simulink model "kin_lin_dyn_FSMRAC_lin2"  (R2017b)
settings: Solver=ode45  StartTime=0.0  StopTime=25  RelTol=1e-3
values from neighbouring files (symbols this model uses):
  act_theta1 = 0.021281    [FSMRAC_lin2.m]
  act_theta2 = 0.02017    [FSMRAC_lin2.m]
  act_theta3 = 1.2e-4    (= 0.00012)    [FSMRAC_lin2.m]
  act_theta4 = 1.0236    [FSMRAC_lin2.m]
  act_theta5 = 1.0438e-4    (= 0.00010438)    [FSMRAC_lin2.m]
  act_theta6 = 1.00271    [FSMRAC_lin2.m]
  alpha = 1    [FSMRAC_lin2.m]
  am = 5    [FSMRAC_lin2.m]
  Am = -am*eye(2)    [FSMRAC_lin2.m]
  Bm = eye(2)    [FSMRAC_lin2.m]
  Cm = eye(2)    [FSMRAC_lin2.m]
  disturbance = 1    [FSMRAC_lin2.m]
  Dm = zeros(2,2)    [FSMRAC_lin2.m]
  Gamma = eye(8)    [FSMRAC_lin2.m]
  P0 = eye(6)    [FSMRAC_lin2.m]
  P_lyap = lyap(Am,Q)    [FSMRAC_lin2.m]
  phi_init = pi/2    (= 1.57079632679)    [FSMRAC_lin2.m]
  R = 2    [FSMRAC_lin2.m]    (also in kinsim.m)
  theta0_c = ones(1,8)    [FSMRAC_lin2.m]
  theta0_m = ones(1,6)    [FSMRAC_lin2.m]
  x_init = 2    [FSMRAC_lin2.m]
  y_init = 0    [FSMRAC_lin2.m]
undefined symbols (not defined in the file or in its folder): magnitude
libraries: simulink_extras x8
settings Model: Creator=nadimkhairallah  LastModifiedBy=nadimkhairallah

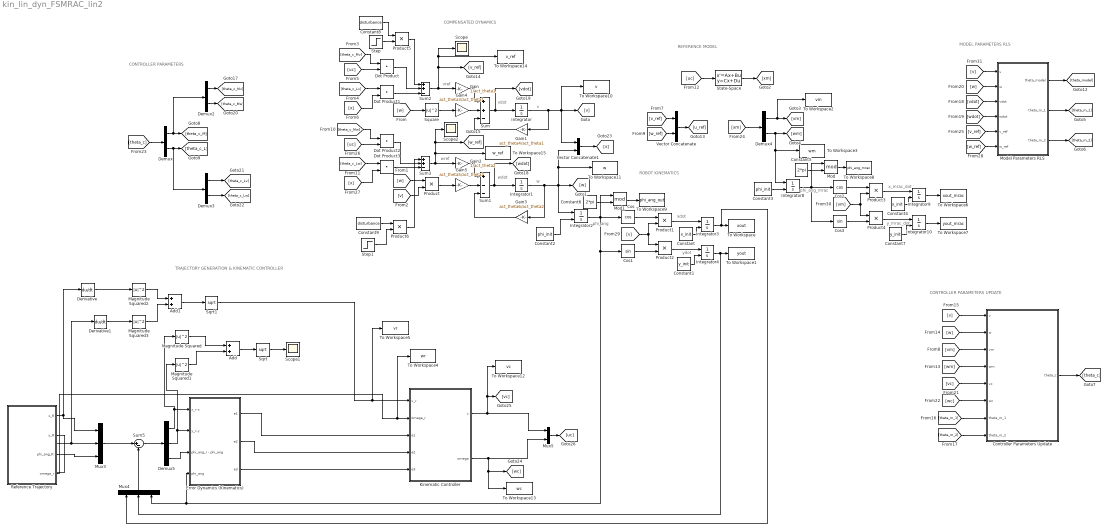
== system kin_lin_dyn_FSMRAC_lin2 ==
  note: ROBOT KINEMATICS
  note: xdot
  note: phi_ang
  note: REFERENCE MODEL
  note: COMPENSATED DYNAMICS
  note: TRAJECTORY GENERATION & KINEMATIC CONTROLLER
  note: CONTROLLER PARAMETERS
  note: w
  note: v
  note: vdot
  note: vref
  note: wdot
  note: wref
  note: CONTROLLER PARAMETERS UPDATE
  note: MODEL PARAMETERS RLS
  note: ydot
  note: y_mrac_dot
  note: x_mrac_dot
  note: phi_ang_mrac
  Add : Sum
  Add1 : Sum
  Constant : Constant  Value=x_init
  Constant1 : Constant  Value=y_init
  Constant2 : Constant  Value=phi_init
  Constant3 : Constant  Value=phi_init
  Constant4 : Constant  Value=x_init
  Constant5 : Constant  Value=2*pi
  Constant6 : Constant  Value=2*pi
  Constant7 : Constant  Value=y_init
  Constant8 : Constant  Value=disturbance
  Constant9 : Constant  Value=disturbance
  Controller Parameters Update : Subsystem
  Cos : Trigonometry  Operator=cos
  Cos1 : Trigonometry
  Cos2 : Trigonometry  Operator=cos
  Cos3 : Trigonometry
  Demux{,2..4} (4 alike) : Demux  Outputs=2
  Demux5 : Demux  Outputs=3
  Derivative : Derivative
  Derivative1 : Derivative
  Dot Product{,1..3} (4 alike) : DotProduct  InputSameDT=on  OutDataTypeStr=Inherit: Inherit via internal rule
  Error Dynamics (Kinematics) : Subsystem
  Gain : Gain  Gain=1/act_theta1
  Gain1 : Gain  Gain=act_theta4/act_theta1
  Gain2 : Gain  Gain=1/act_theta2
  Gain3 : Gain  Gain=act_theta6/act_theta2
  Gain4 : Gain  Gain=act_theta3/act_theta1
  Gain5 : Gain  Gain=act_theta5/act_theta2
  Integrator : Integrator
  Integrator1 : Integrator
  Integrator{2..4,8..10} (6 alike) : Integrator  InitialConditionSource=external
  Kinematic Controller : Subsystem
  Magnitude Squared{,1..3} (4 alike) : Math  Operator=magnitude^2  SaturateOnIntegerOverflow=on
  Mod : Math  Operator=mod  SaturateOnIntegerOverflow=on
  Mod1 : Math  Operator=mod  SaturateOnIntegerOverflow=on
  Model Parameters RLS : Subsystem
  Mux3 : Mux  Inputs=3
  Mux4 : Mux  Inputs=3
  Mux5 : Mux  Inputs=2
  Product{,1..6} (7 alike) : Product
  Reference Trajectory : Subsystem
  Scope : Scope
  Scope1 : Scope
  Scope2 : Scope
  Sqrt : Sqrt  SaturateOnIntegerOverflow=on
  Sqrt1 : Sqrt  SaturateOnIntegerOverflow=on
  Square : Math  Operator=magnitude^2  RndMeth=Zero  SaturateOnIntegerOverflow=on
  State-Space : StateSpace  A=Am  B=Bm  C=Cm  D=Dm  InitialCondition=0
  Step : Step  Time=15  After=0.5  SampleTime=0
  Step1 : Step  Time=10  After=0.5  SampleTime=0
  Sum : Sum  Inputs=++-
  Sum1 : Sum  Inputs=+--
  Sum2 : Sum  Inputs=++-
  Sum3 : Sum  Inputs=++-
  Sum5 : Sum  Inputs=|+-
  To Workspace : ToWorkspace  VariableName=xout  SampleTime=-1
      settings: Save2DSignal=2-D array (concatenate along first dimension)
  To Workspace1 : ToWorkspace  VariableName=yout  SampleTime=-1
      settings: Save2DSignal=2-D array (concatenate along first dimension)
  To Workspace10 : ToWorkspace  VariableName=v  SampleTime=-1
  To Workspace11 : ToWorkspace  VariableName=w  SampleTime=-1
  To Workspace12 : ToWorkspace  VariableName=vc  SampleTime=-1
      settings: Save2DSignal=2-D array (concatenate along first dimension)
  To Workspace13 : ToWorkspace  VariableName=wc  SampleTime=-1
      settings: Save2DSignal=2-D array (concatenate along first dimension)
  To Workspace14 : ToWorkspace  VariableName=v_ref  SampleTime=-1
  To Workspace15 : ToWorkspace  VariableName=w_ref  SampleTime=-1
  To Workspace2 : ToWorkspace  VariableName=vm  SampleTime=-1
  To Workspace3 : ToWorkspace  VariableName=wm  SampleTime=-1
  To Workspace4 : ToWorkspace  VariableName=wr  SampleTime=-1
  To Workspace5 : ToWorkspace  VariableName=vr  SampleTime=-1
  To Workspace6 : ToWorkspace  VariableName=xout_mrac  SampleTime=-1
  To Workspace7 : ToWorkspace  VariableName=yout_mrac  SampleTime=-1
  To Workspace8 : ToWorkspace  VariableName=phi_ang_mrac  SampleTime=-1
  To Workspace9 : ToWorkspace  VariableName=phi_ang_out  SampleTime=-1
      settings: Save2DSignal=2-D array (concatenate along first dimension)
  Vector Concatenate : Concatenate
  Vector Concatenate1 : Concatenate
  wires:
  Gain/1 -> Sum/1
  Gain1/1 -> Sum/3
  Gain3/1 -> Sum1/3
  Gain2/1 -> Sum1/1
  [w] -> Square/1
  Gain4/1 -> Sum/2
  Square/1 -> Gain4/1
  Gain5/1 -> Sum1/2
  Product/1 -> Gain5/1
  [w] -> Product/1
  [v] -> Product/2
  [v] -> Controller Parameters Update/1(v)
  [w] -> Controller Parameters Update/2(w)
  [vm] -> Controller Parameters Update/3(vm)
  [wm] -> Controller Parameters Update/4(wm)
  [theta_m_1] -> Controller Parameters Update/7(theta_m_1)
  [theta_m_2] -> Controller Parameters Update/8(theta_m_2)
  [vc] -> Controller Parameters Update/5(vc)
  [wc] -> Controller Parameters Update/6(wc)
  Controller Parameters Update/1(theta_c) -> [theta_c]
  [theta_c] -> Demux/1
  Demux/1 -> [theta_c_M], Demux2/1
  Demux/2 -> Demux3/1, [theta_c_L]
  Demux2/1 -> [theta_c_Mv]
  Demux2/2 -> [theta_c_Mw]
  Demux3/1 -> [theta_c_Lv]
  Demux3/2 -> [theta_c_Lw]
  [theta_c_Mv] -> Dot Product/1
  [uc] -> Dot Product/2
  [theta_c_Lv] -> Dot Product1/1
  [x] -> Dot Product1/2
  [v_ref] -> Vector Concatenate/1
  Vector Concatenate/1 -> [u_ref]
  [x] -> Dot Product3/2
  [theta_c_Lw] -> Dot Product3/1
  [uc] -> Dot Product2/2
  [theta_c_Mw] -> Dot Product2/1
  [uc] -> State-Space/1
  State-Space/1 -> [xm]
  [xm] -> Demux4/1
  Demux4/1 -> To Workspace2/1, [vm]
  Demux4/2 -> Integrator8/1, To Workspace3/1, [wm]
  [w_ref] -> Vector Concatenate/2
  Vector Concatenate1/1 -> [x]
  [vdot] -> Model Parameters RLS/3("vdot ")
  Model Parameters RLS/1(theta_model) -> [theta_model]
  [w] -> Model Parameters RLS/2(w)
  [v] -> Model Parameters RLS/1(v)
  [wdot] -> Model Parameters RLS/4("wdot ")
  [v_ref] -> Model Parameters RLS/5(v_ref)
  Model Parameters RLS/2(theta_m_1) -> [theta_m_1]
  Model Parameters RLS/3(theta_m_2) -> [theta_m_2]
  [w_ref] -> Model Parameters RLS/6(w_ref)
  Integrator1/1 -> [w], Integrator2/1, To Workspace11/1, Vector Concatenate1/2, Gain3/1
  Sum/1 -> [vdot], Integrator/1
  Sum1/1 -> [wdot], Integrator1/1
  Sum2/1 -> Scope/1, To Workspace14/1, [v_ref], Gain/1
  Sum3/1 -> To Workspace15/1, [w_ref], Scope2/1, Gain2/1
  Cos/1 -> Product1/1
  [v] -> Product2/1, Product1/2
  Cos1/1 -> Product2/2
  Product1/1 -> Integrator3/1
  Product2/1 -> Integrator4/1
  Constant/1 -> Integrator3/2
  Constant1/1 -> Integrator4/2
  Constant2/1 -> Integrator2/2
  Magnitude Squared2/1 -> Add1/1
  Magnitude Squared3/1 -> Add1/2
  Reference Trajectory/3("phi_ang_R ") -> Mux3/3
  Derivative1/1 -> Magnitude Squared3/1
  Reference Trajectory/1("x_R ") -> Mux3/1, Derivative/1
  Integrator3/1 -> Mux4/1, To Workspace/1
  Mux3/1 -> Sum5/1
  Add/1 -> Sqrt/1
  Magnitude Squared1/1 -> Add/2
  Error Dynamics (Kinematics)/2(e2) -> Kinematic Controller/4(e2)
  Error Dynamics (Kinematics)/3(e3) -> Kinematic Controller/5(e3)
  Integrator4/1 -> Mux4/2, To Workspace1/1
  Sum5/1 -> Demux5/1
  Sqrt/1 -> Scope1/1
  Mux4/1 -> Sum5/2
  Magnitude Squared/1 -> Add/1
  Demux5/3 -> Error Dynamics (Kinematics)/3("phi_ang_r - phi_ang ")
  Reference Trajectory/4("omega_r ") -> To Workspace4/1, Kinematic Controller/2(omega_r)
  Integrator2/1 -> Mod1/1, Mux4/3, Error Dynamics (Kinematics)/4(phi_ang), Cos1/1, Cos/1
  Error Dynamics (Kinematics)/1(e1) -> Kinematic Controller/3(e1)
  Demux5/2 -> Magnitude Squared1/1, Error Dynamics (Kinematics)/2(y_r-y)
  Add1/1 -> Sqrt1/1
  Demux5/1 -> Magnitude Squared/1, Error Dynamics (Kinematics)/1("x_r-x ")
  Derivative/1 -> Magnitude Squared2/1
  Reference Trajectory/2("y_R ") -> Derivative1/1, Mux3/2
  Sqrt1/1 -> Kinematic Controller/1(v_r), To Workspace5/1
  Mux5/1 -> [uc]
  Kinematic Controller/2(omega) -> To Workspace13/1, [wc], Mux5/2
  Kinematic Controller/1(v) -> Mux5/1, To Workspace12/1, [vc]
  Cos3/1 -> Product4/2
  Cos2/1 -> Product3/1
  Constant3/1 -> Integrator8/2
  Constant7/1 -> Integrator10/2
  Integrator10/1 -> To Workspace7/1
  Product4/1 -> Integrator10/1
  [vm] -> Product3/2, Product4/1
  Constant4/1 -> Integrator9/2
  Product3/1 -> Integrator9/1
  Integrator9/1 -> To Workspace6/1
  Mod/1 -> To Workspace8/1
  Integrator8/1 -> Mod/1, Cos2/1, Cos3/1
  Constant5/1 -> Mod/2
  Constant6/1 -> Mod1/2
  Mod1/1 -> To Workspace9/1
  Integrator/1 -> [v], Vector Concatenate1/1, To Workspace10/1, Gain1/1
  Dot Product1/1 -> Sum2/3
  Dot Product/1 -> Sum2/2
  Dot Product3/1 -> Sum3/3
  Dot Product2/1 -> Sum3/2
  Step/1 -> Product5/2
  Constant8/1 -> Product5/1
  Product5/1 -> Sum2/1
  Constant9/1 -> Product6/1
  Step1/1 -> Product6/2
  Product6/1 -> Sum3/1

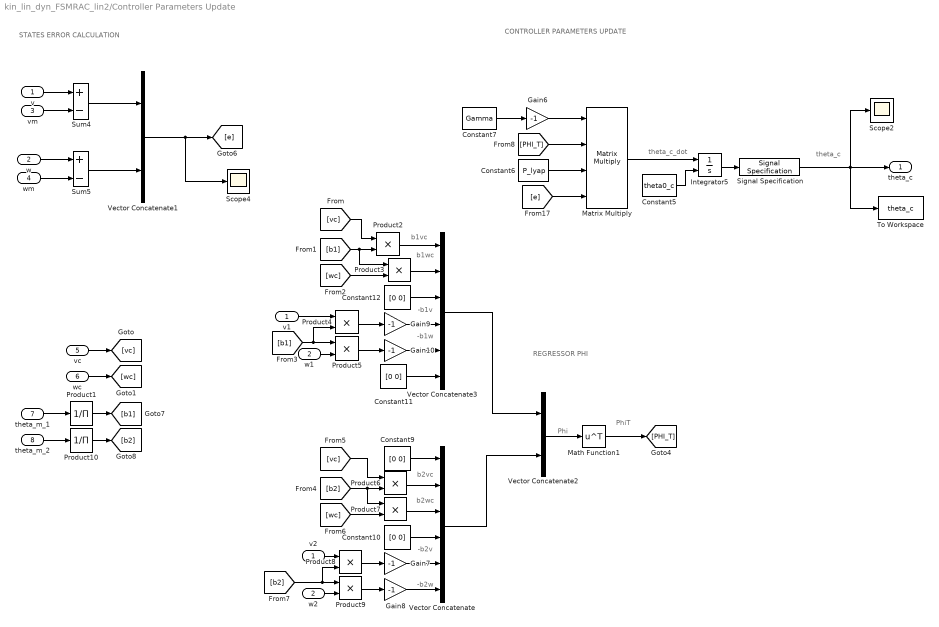
== system kin_lin_dyn_FSMRAC_lin2/Controller Parameters Update ==
  note: -b2v
  note: b2vc
  note: theta_c
  note: theta_c_dot
  note: STATES ERROR CALCULATION
  note: CONTROLLER PARAMETERS UPDATE
  note: PhiT
  note: REGRESSOR PHI
  note: Phi
  note: b2wc
  note: -b2w
  note: b1vc
  note: b1wc
  note: -b1v
  note: -b1w
  v : Inport
  w : Inport  Port=2
  vm : Inport  Port=3
  wm : Inport  Port=4
  vc : Inport  Port=5
  wc : Inport  Port=6
  theta_m_1 : Inport  Port=7
  theta_m_2 : Inport  Port=8
  Constant{9..12} (4 alike) : Constant  Value=[0 0]  VectorParams1D=off
  Constant5 : Constant  Value=theta0_c
  Constant6 : Constant  Value=P_lyap  VectorParams1D=off
  Constant7 : Constant  Value=Gamma  VectorParams1D=off
  Gain{6..10} (5 alike) : Gain  Gain=-1
  Integrator5 : Integrator  InitialConditionSource=external
  Math Function1 : Math  Operator=transpose  SaturateOnIntegerOverflow=on
  Matrix Multiply : Product  Inputs=4  Multiplication=Matrix(*)
  Product1 : Product  Inputs=/
  Product10 : Product  Inputs=/
  Product{2..9} (8 alike) : Product
  Scope2 : Scope
  Scope4 : Scope
  Signal Specification : SignalSpecification  Dimensions=8*1
  Sum4 : Sum  Inputs=+-
  Sum5 : Sum  Inputs=+-
  To Workspace : ToWorkspace  VariableName=theta_c  SampleTime=-1
      settings: Save2DSignal=2-D array (concatenate along first dimension)
  Vector Concatenate : Concatenate  NumInputs=6
  Vector Concatenate1 : Concatenate  Mode=Multidimensional array
  Vector Concatenate2 : Concatenate  Mode=Multidimensional array
  Vector Concatenate3 : Concatenate  NumInputs=6
  v1 : InportShadow
  v2 : InportShadow
  w1 : InportShadow  Port=2
  w2 : InportShadow  Port=2
  theta_c : Outport
  wires:
  Constant10/1 -> Vector Concatenate/4
  Gain8/1 -> Vector Concatenate/6
  Vector Concatenate2/1 -> Math Function1/1
  Gain6/1 -> Matrix Multiply/1
  Constant12/1 -> Vector Concatenate3/3
  Sum4/1 -> Vector Concatenate1/1
  [e] -> Matrix Multiply/4
  Constant11/1 -> Vector Concatenate3/6
  Constant6/1 -> Matrix Multiply/3
  Vector Concatenate3/1 -> Vector Concatenate2/1
  Math Function1/1 -> [PHI_T]
  Constant7/1 -> Gain6/1
  Sum5/1 -> Vector Concatenate1/2
  Gain10/1 -> Vector Concatenate3/5
  Gain9/1 -> Vector Concatenate3/4
  Matrix Multiply/1 -> Integrator5/1
  Constant5/1 -> Integrator5/2
  Vector Concatenate/1 -> Vector Concatenate2/2
  [PHI_T] -> Matrix Multiply/2
  Constant9/1 -> Vector Concatenate/1
  Vector Concatenate1/1 -> [e], Scope4/1
  Gain7/1 -> Vector Concatenate/5
  v/1 -> Sum4/1
  w/1 -> Sum5/1
  wm/1 -> Sum5/2
  vm/1 -> Sum4/2
  vc/1 -> [vc]
  wc/1 -> [wc]
  Product2/1 -> Vector Concatenate3/1
  [vc] -> Product2/1
  [b1] -> Product3/1, Product2/2
  Product3/1 -> Vector Concatenate3/2
  [wc] -> Product3/2
  Product4/1 -> Gain9/1
  Product5/1 -> Gain10/1
  v1/1 -> Product4/1
  [b1] -> Product4/2, Product5/1
  w1/1 -> Product5/2
  Product6/1 -> Vector Concatenate/2
  Product7/1 -> Vector Concatenate/3
  [b2] -> Product7/1, Product6/2
  [vc] -> Product6/1
  [wc] -> Product7/2
  Product8/1 -> Gain7/1
  Product9/1 -> Gain8/1
  v2/1 -> Product8/1
  [b2] -> Product8/2, Product9/1
  w2/1 -> Product9/2
  theta_m_2/1 -> Product10/1
  theta_m_1/1 -> Product1/1
  Product1/1 -> [b1]
  Product10/1 -> [b2]
  Integrator5/1 -> Signal Specification/1
  Signal Specification/1 -> To Workspace/1, Scope2/1, theta_c/1

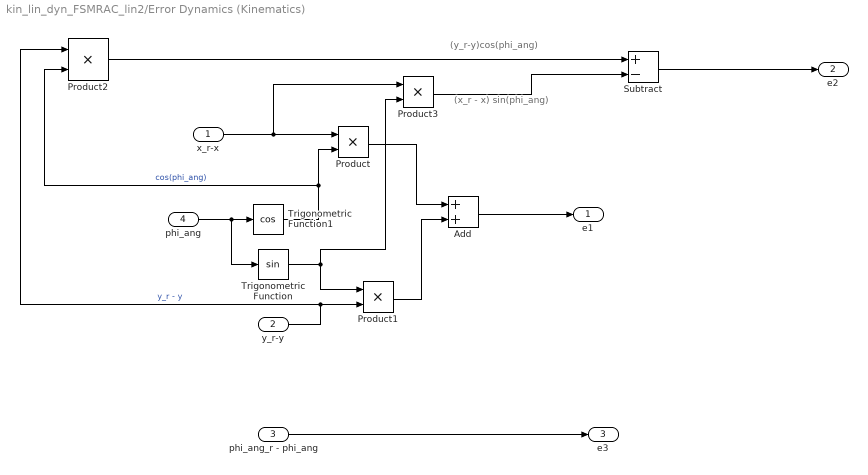
== system kin_lin_dyn_FSMRAC_lin2/Error Dynamics (Kinematics) ==
  note: (x_r - x) sin(phi_ang)
  note: (y_r-y)cos(phi_ang)
  "x_r-x " : Inport
  y_r-y : Inport  Port=2
  "phi_ang_r - phi_ang " : Inport  Port=3
  phi_ang : Inport  Port=4
  Add : Sum
  Product{,1..3} (4 alike) : Product
  Subtract : Sum  Inputs=+-
  Trigonometric Function : Trigonometry
  Trigonometric Function1 : Trigonometry  Operator=cos
  e1 : Outport  VectorParamsAs1DForOutWhenUnconnected=on
  e2 : Outport  Port=2  VectorParamsAs1DForOutWhenUnconnected=on
  e3 : Outport  Port=3  VectorParamsAs1DForOutWhenUnconnected=on
  wires:
  "x_r-x "/1 -> Product3/1, Product/1
  phi_ang/1 -> Trigonometric Function/1, Trigonometric Function1/1
  Trigonometric Function1/1 -> Product2/2, Product/2  "cos(phi_ang)"
  Trigonometric Function/1 -> Product3/2, Product1/1
  y_r-y/1 -> Product2/1, Product1/2  "y_r - y"
  "phi_ang_r - phi_ang "/1 -> e3/1
  Product1/1 -> Add/2
  Product/1 -> Add/1
  Add/1 -> e1/1
  Product2/1 -> Subtract/1
  Product3/1 -> Subtract/2
  Subtract/1 -> e2/1

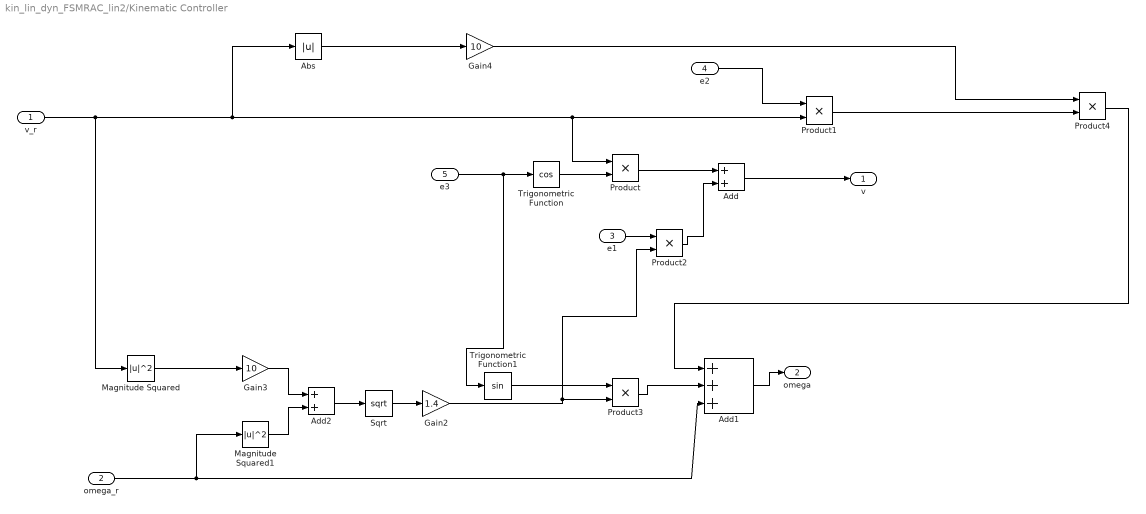
== system kin_lin_dyn_FSMRAC_lin2/Kinematic Controller ==
  v_r : Inport
  omega_r : Inport  Port=2
  e1 : Inport  Port=3
  e2 : Inport  Port=4
  e3 : Inport  Port=5
  Abs : Abs
  Add : Sum
  Add1 : Sum  Inputs=+++
  Add2 : Sum
  Gain2 : Gain  Gain=1.4
  Gain3 : Gain  Gain=10
  Gain4 : Gain  Gain=10
  Magnitude Squared : Math  Operator=magnitude^2  SaturateOnIntegerOverflow=on
  Magnitude Squared1 : Math  Operator=magnitude^2  SaturateOnIntegerOverflow=on
  Product{,1..4} (5 alike) : Product
  Sqrt : Sqrt  SaturateOnIntegerOverflow=on
  Trigonometric Function : Trigonometry  Operator=cos
  Trigonometric Function1 : Trigonometry
  v : Outport  VectorParamsAs1DForOutWhenUnconnected=on
  omega : Outport  Port=2  VectorParamsAs1DForOutWhenUnconnected=on
  wires:
  Trigonometric Function/1 -> Product/2
  v_r/1 -> Abs/1, Product/1, Product1/2, Magnitude Squared/1
  Product/1 -> Add/1
  e1/1 -> Product2/1
  Product2/1 -> Add/2
  Add/1 -> v/1
  Add1/1 -> omega/1
  Trigonometric Function1/1 -> Product3/1
  e3/1 -> Trigonometric Function1/1, Trigonometric Function/1
  omega_r/1 -> Add1/3, Magnitude Squared1/1
  Product3/1 -> Add1/2
  Product4/1 -> Add1/1
  e2/1 -> Product1/1
  Product1/1 -> Product4/2
  Magnitude Squared1/1 -> Add2/2
  Magnitude Squared/1 -> Gain3/1
  Gain3/1 -> Add2/1
  Add2/1 -> Sqrt/1
  Sqrt/1 -> Gain2/1
  Gain2/1 -> Product2/2, Product3/2
  Abs/1 -> Gain4/1
  Gain4/1 -> Product4/1

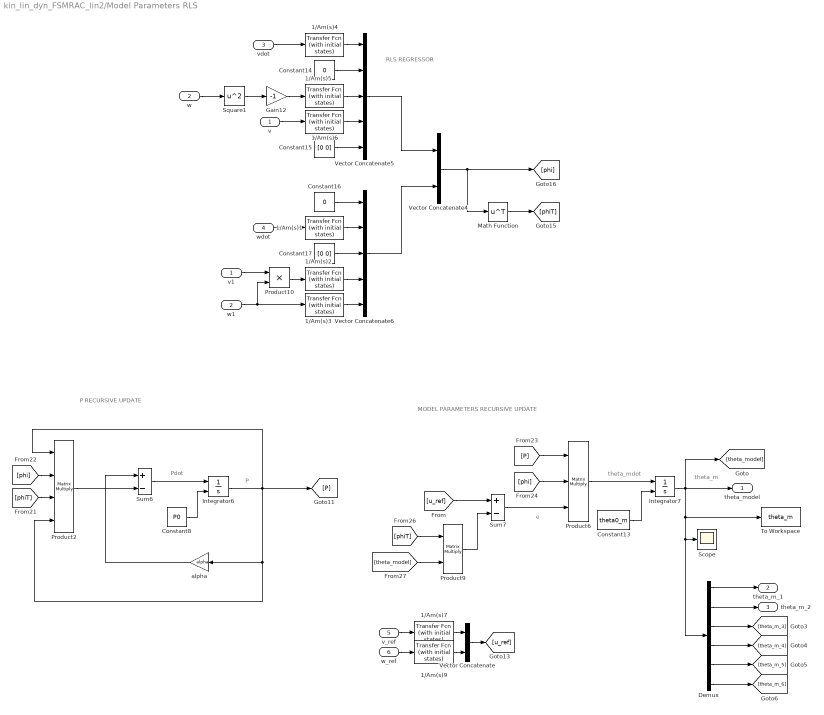
== system kin_lin_dyn_FSMRAC_lin2/Model Parameters RLS ==
  note: e
  note: theta_m
  note: theta_mdot
  note: P
  note: Pdot
  note: MODEL PARAMETERS RECURSIVE UPDATE
  note: P RECURSIVE UPDATE
  note: RLS REGRESSOR
  v : Inport  PortDimensions=1
  w : Inport  Port=2  PortDimensions=1
  "vdot " : Inport  Port=3  PortDimensions=1
  "wdot " : Inport  Port=4  PortDimensions=1
  v_ref : Inport  Port=5  PortDimensions=1
  w_ref : Inport  Port=6  PortDimensions=1
  1/Am(s){1..7,9} (8 alike) : simulink_extras/Additional Linear/Transfer Fcn (with initial states)  N=[1]  D=[1 2*am am^2]  X0=.5
  Constant13 : Constant  Value=theta0_m
  Constant14 : Constant  Value=0
  Constant15 : Constant  Value=[0 0]
  Constant16 : Constant  Value=0
  Constant17 : Constant  Value=[0 0]
  Constant8 : Constant  Value=P0
  Demux : Demux  Outputs=6
  Gain12 : Gain  Gain=-1
  Integrator6 : Integrator  InitialConditionSource=external  InitialCondition=P0
  Integrator7 : Integrator  InitialConditionSource=external  InitialCondition=P0
  Math Function : Math  Operator=transpose  SaturateOnIntegerOverflow=on
  Product10 : Product
  Product2 : Product  Inputs=4  Multiplication=Matrix(*)
  Product6 : Product  Inputs=3  Multiplication=Matrix(*)
  Product9 : Product  Multiplication=Matrix(*)
  Scope : Scope
  Square1 : Math  Operator=square  RndMeth=Zero  SaturateOnIntegerOverflow=on
  Sum6 : Sum  Inputs=+-
  Sum7 : Sum  Inputs=+-
  To Workspace : ToWorkspace  VariableName=theta_m  SampleTime=-1
  Vector Concatenate : Concatenate
  Vector Concatenate4 : Concatenate  Mode=Multidimensional array  ConcatenateDimension=2
  Vector Concatenate5 : Concatenate  NumInputs=5  ConcatenateDimension=2
  Vector Concatenate6 : Concatenate  NumInputs=5  ConcatenateDimension=2
  "alpha " : Gain  Gain=alpha
  v1 : InportShadow  PortDimensions=1
  w1 : InportShadow  Port=2  PortDimensions=1
  theta_model : Outport
  theta_m_1 : Outport  Port=2
  theta_m_2 : Outport  Port=3
  wires:
  Constant15/1 -> Vector Concatenate5/5
  Constant17/1 -> Vector Concatenate6/3
  1/Am(s)5/1 -> Vector Concatenate5/3
  1/Am(s)2/1 -> Vector Concatenate6/4
  Gain12/1 -> 1/Am(s)5/1
  Product10/1 -> 1/Am(s)2/1
  1/Am(s)3/1 -> Vector Concatenate6/5
  Vector Concatenate5/1 -> Vector Concatenate4/1
  1/Am(s)4/1 -> Vector Concatenate5/1
  [phiT] -> Product9/1
  [theta_model] -> Product9/2
  Constant13/1 -> Integrator7/2
  Integrator6/1 -> Product2/4, "alpha "/1, [P], Product2/1
  [phi] -> Product2/2
  Sum7/1 -> Product6/3
  Product6/1 -> Integrator7/1
  Math Function/1 -> [phiT]
  "alpha "/1 -> Sum6/1
  [phiT] -> Product2/3
  Vector Concatenate4/1 -> Math Function/1, [phi]
  Sum6/1 -> Integrator6/1
  Constant8/1 -> Integrator6/2
  Product2/1 -> Sum6/2
  Integrator7/1 -> [theta_model], theta_model/1, To Workspace/1, Scope/1, Demux/1
  Product9/1 -> Sum7/2
  [phi] -> Product6/2
  [P] -> Product6/1
  w1/1 -> 1/Am(s)3/1, Product10/2
  Constant16/1 -> Vector Concatenate6/1
  Square1/1 -> Gain12/1
  Vector Concatenate6/1 -> Vector Concatenate4/2
  1/Am(s)6/1 -> Vector Concatenate5/4
  1/Am(s)1/1 -> Vector Concatenate6/2
  Constant14/1 -> Vector Concatenate5/2
  v/1 -> 1/Am(s)6/1
  v1/1 -> Product10/1
  w/1 -> Square1/1
  "vdot "/1 -> 1/Am(s)4/1
  "wdot "/1 -> 1/Am(s)1/1
  Demux/3 -> [theta_m_3]
  Demux/4 -> [theta_m_4]
  Demux/5 -> [theta_m_5]
  Demux/6 -> [theta_m_6]
  Demux/2 -> theta_m_2/1
  Demux/1 -> theta_m_1/1
  w_ref/1 -> 1/Am(s)9/1
  v_ref/1 -> 1/Am(s)7/1
  Vector Concatenate/1 -> [u_ref]
  [u_ref] -> Sum7/1
  1/Am(s)7/1 -> Vector Concatenate/1
  1/Am(s)9/1 -> Vector Concatenate/2

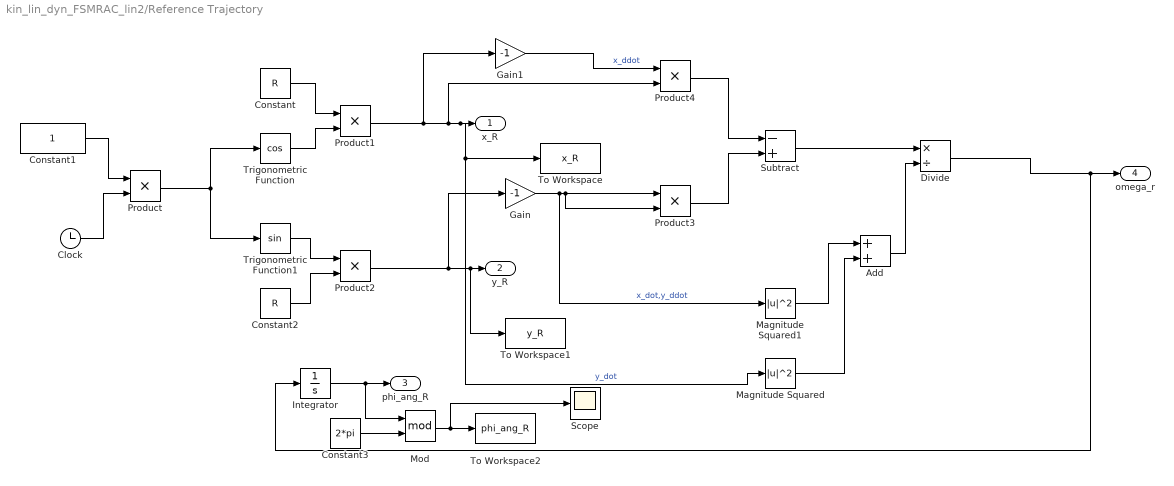
== system kin_lin_dyn_FSMRAC_lin2/Reference Trajectory ==
  Add : Sum
  Clock : Clock
  Constant : Constant  Value=R
  Constant1 : Constant
  Constant2 : Constant  Value=R
  Constant3 : Constant  Value=2*pi
  Divide : Product  Inputs=*/
  Gain : Gain  Gain=-1
  Gain1 : Gain  Gain=-1
  Integrator : Integrator
  Magnitude Squared : Math  Operator=magnitude^2  SaturateOnIntegerOverflow=on
  Magnitude Squared1 : Math  Operator=magnitude^2  SaturateOnIntegerOverflow=on
  Mod : Math  Operator=mod  SaturateOnIntegerOverflow=on
  Product{,1..4} (5 alike) : Product
  Scope : Scope
  Subtract : Sum  Inputs=-+
  To Workspace : ToWorkspace  VariableName=x_R  SampleTime=-1
  To Workspace1 : ToWorkspace  VariableName=y_R  SampleTime=-1
  To Workspace2 : ToWorkspace  VariableName=phi_ang_R  SampleTime=-1
  Trigonometric Function : Trigonometry  Operator=cos
  Trigonometric Function1 : Trigonometry
  "x_R " : Outport  VectorParamsAs1DForOutWhenUnconnected=on
  "y_R " : Outport  Port=2  VectorParamsAs1DForOutWhenUnconnected=on
  "phi_ang_R " : Outport  Port=3  VectorParamsAs1DForOutWhenUnconnected=on
  "omega_r " : Outport  Port=4  VectorParamsAs1DForOutWhenUnconnected=on
  wires:
  Product1/1 -> Gain1/1, To Workspace/1, Magnitude Squared/1, "x_R "/1, Product4/2  "y_dot"
  Clock/1 -> Product/2
  Integrator/1 -> Mod/1, "phi_ang_R "/1
  Constant1/1 -> Product/1
  Constant2/1 -> Product2/2
  Trigonometric Function/1 -> Product1/2
  Constant/1 -> Product1/1
  Product2/1 -> Gain/1, To Workspace1/1, "y_R "/1
  Product/1 -> Trigonometric Function1/1, Trigonometric Function/1
  Trigonometric Function1/1 -> Product2/1
  Gain/1 -> Magnitude Squared1/1, Product3/2, Product3/1  "x_dot,y_ddot"
  Gain1/1 -> Product4/1  "x_ddot"
  Product3/1 -> Subtract/2
  Product4/1 -> Subtract/1
  Subtract/1 -> Divide/1
  Add/1 -> Divide/2
  Magnitude Squared1/1 -> Add/1
  Magnitude Squared/1 -> Add/2
  Divide/1 -> Integrator/1, "omega_r "/1
  Mod/1 -> Scope/1, To Workspace2/1
  Constant3/1 -> Mod/2
